simulink library "INT_PTODi_TrqDesCoord"  (R2016b)
settings: Solver=VariableStepAuto  StartTime=0.0  StopTime=10.0  RelTol=1e-3
settings Model: Creator=Administrator  LastModifiedBy=Administrator

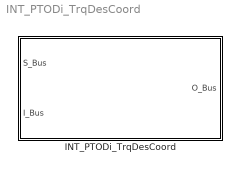
== system INT_PTODi_TrqDesCoord ==
  INT_PTODi_TrqDesCoord : Subsystem

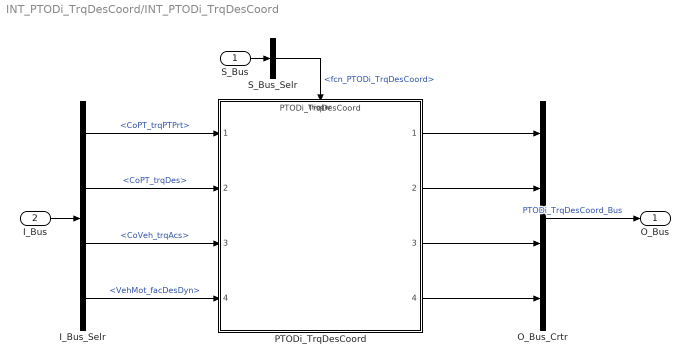
== system INT_PTODi_TrqDesCoord/INT_PTODi_TrqDesCoord ==
  S_Bus : Inport
  I_Bus : Inport  Port=2
  I_Bus_Selr : BusSelector  OutputSignals=CoPT_trqPTPrt,CoPT_trqDes,CoVeh_trqAcs,VehMot_facDesDyn
  O_Bus_Crtr : BusCreator  Inputs=4
  PTODi_TrqDesCoord : ModelReference  ModelNameDialog=PTODi_TrqDesCoord  SimulationMode=Normal  ModelReferenceVersion=1.8  TriggerPortName=function  TriggerPortTriggerType=function-call  TriggerPortStatesWhenEnabling=held
  S_Bus_Selr : BusSelector  OutputSignals=fcn_PTODi_TrqDesCoord
  O_Bus : Outport
  wires:
  S_Bus_Selr/1 -> PTODi_TrqDesCoord/Trigger  "<fcn_PTODi_TrqDesCoord>"
  S_Bus/1 -> S_Bus_Selr/1
  I_Bus/1 -> I_Bus_Selr/1
  I_Bus_Selr/1 -> PTODi_TrqDesCoord/1  "<CoPT_trqPTPrt>"
  I_Bus_Selr/2 -> PTODi_TrqDesCoord/2  "<CoPT_trqDes>"
  I_Bus_Selr/3 -> PTODi_TrqDesCoord/3  "<CoVeh_trqAcs>"
  I_Bus_Selr/4 -> PTODi_TrqDesCoord/4  "<VehMot_facDesDyn>"
  O_Bus_Crtr/1 -> O_Bus/1  "PTODi_TrqDesCoord_Bus"
  PTODi_TrqDesCoord/1 -> O_Bus_Crtr/1
  PTODi_TrqDesCoord/2 -> O_Bus_Crtr/2
  PTODi_TrqDesCoord/3 -> O_Bus_Crtr/3
  PTODi_TrqDesCoord/4 -> O_Bus_Crtr/4
